simulink model "simulink_verify"  (R2018a)
settings: Solver=VariableStepAuto  StartTime=0.0  StopTime=100  RelTol=1e-3
model workspace: external: MAT-File /home/owen/Desktop/play_ground/src/system_identification_car/scripts/all_current_space_2.mat (data not in the file)
undefined symbols (not defined in the file or in its folder): K, robust_ss
settings Model: Creator=root  LastModifiedBy=root

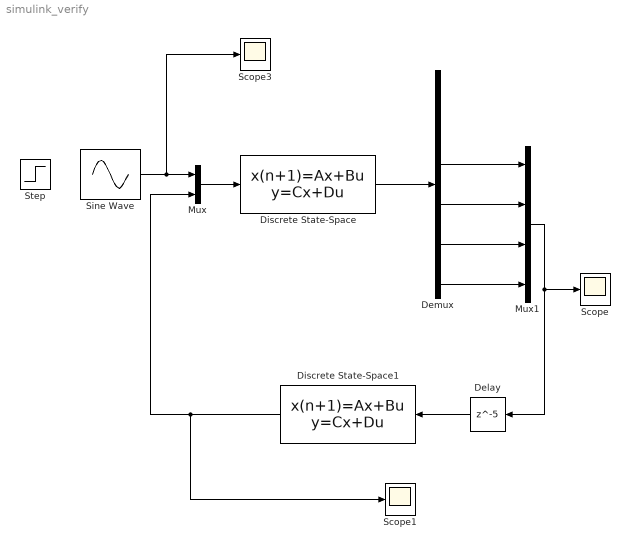
== system simulink_verify ==
  Delay : Delay  DelayLength=5  SampleTime=0.0333
  Demux : Demux  Outputs=6
  Discrete State-Space : DiscreteStateSpace  A=robust_ss.NominalValue.A  B=robust_ss.NominalValue.B  C=robust_ss.C  D=robust_ss.D  SampleTime=0.0333
  Discrete State-Space1 : DiscreteStateSpace  A=K.A  B=K.B  C=K.C  D=K.D  SampleTime=0.0333
  Mux : Mux  Inputs=2
  Mux1 : Mux
  Scope : Scope
  Scope1 : Scope
  Scope3 : Scope
  Sine Wave : Sin  Amplitude=0.5  Frequency=0.1  SampleTime=0.0333
  Step : Step  SampleTime=0
  wires:
  Mux/1 -> Discrete State-Space/1
  Discrete State-Space/1 -> Demux/1
  Demux/3 -> Mux1/1
  Demux/4 -> Mux1/2
  Demux/5 -> Mux1/3
  Demux/6 -> Mux1/4
  Discrete State-Space1/1 -> Mux/2, Scope1/1
  Mux1/1 -> Delay/1, Scope/1
  Sine Wave/1 -> Scope3/1, Mux/1
  Delay/1 -> Discrete State-Space1/1
